simulink model "cube0_mpc_tp_ls"  (R2022b)
settings: Solver=VariableStepAuto  StartTime=0.0  StopTime=1000  RelTol=1e-3  AbsTol=1e-3
libraries: mpclib x1
settings Model: Creator=Abhijit  LastModifiedBy=Abhijit
settings SolverCC: AutoScaleAbsTol=off  AlgebraicLoopSolver=TrustRegion  MaxZcPerStep=1
settings DataIOCC: SaveFormat=StructureWithTime
settings DebuggingCC: UnconnectedInputMsg=warning  UnconnectedOutputMsg=warning  UnconnectedLineMsg=warning  SymbolicDimsDataTypeCodeGenerationDiagnostic=none  SFMachineParentedDataDiag=warning
settings ModelReferenceCC: EnableRefExpFcnMdlSchedulingChecks=on
settings SFSimCC: CustomCodeUndefinedFunction=UseInterfaceOnly
settings RTWCC: DLArmComputeVersion=19.05
settings SimscapeCC: SimscapeLogType=all  SimscapeLogSimulationStatistics=on  SimscapeLogDataHistory=10000

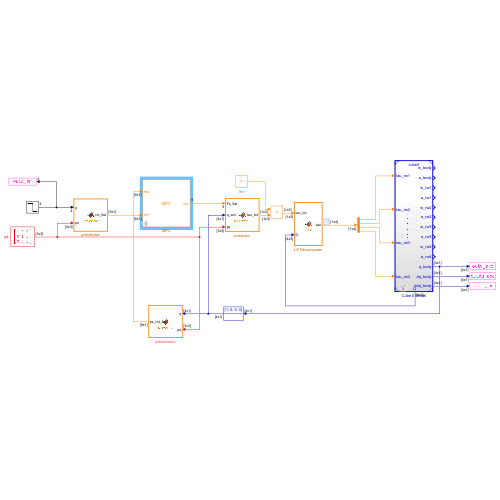
[thumbnail: Simulink's stored preview of the top-level diagram]
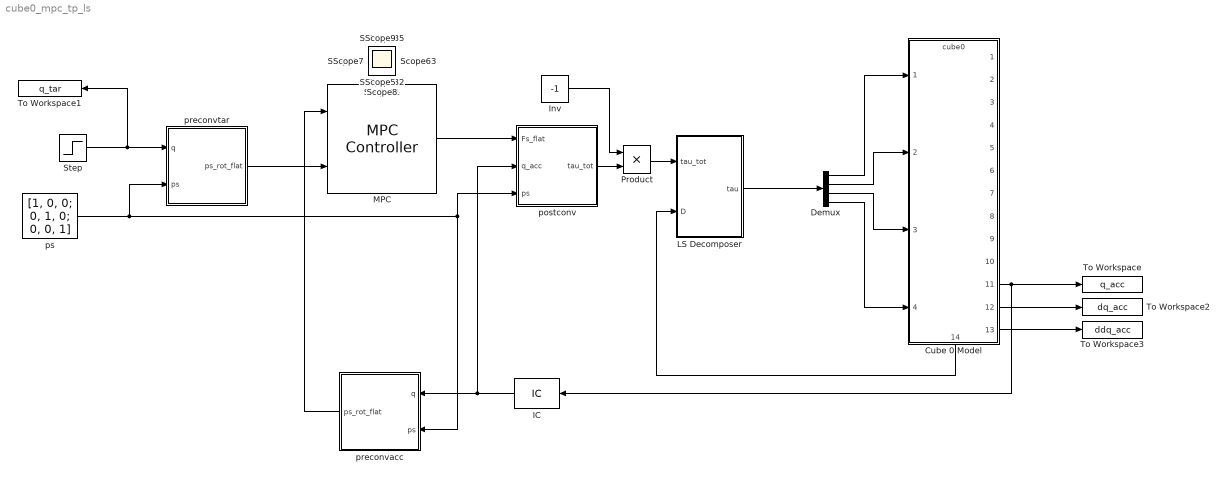
== system cube0_mpc_tp_ls ==
  Cube 0 Model : ModelReference  ModelNameDialog=cube0.slx  SimulationMode=Normal  ModelReferenceVersion=1.7
      settings: PortSchema="{\"entries\":[{\"content\":{\"sides\":[{\"content\":{\"connectorIds\":[\"In1\",\"In2\",\"In3\",\"In4\"]},\"type\":\"ConnectorPlacement.EquallySpacedRectSide\",\"uuid\":\"8e9d2764-0c8c-4b35-a6b5-330d2d8aade7\"},{\"content\":{\"connectorIds\":[\"Out1\",\"Out2\",\"Out3\",\"Out4\",\"Out5\",\"Out6\",\"Out7\",\"Out8\",\"Out9\",\"Out10\",\"Out11\",\"Out12\",\"Out13\"],\"side\":\"RIGHT\"},\"type\":\"ConnectorPlacement.EquallySpacedRectSide\",\"uuid\":\"d11583f7-9081-4803-9c4e-bf58094124c2\"},{\"content\":{\"connectorIds\":[],\"side\":\"TOP\"},\"type\":\"ConnectorPlacement.EquallySpacedRectSide\",\"uuid\":\"f987c09c-5813-428e-a812-016ca0940eea\"},{\"content\":{\"connectorIds\":[\"Out14\"],\"side\":\"BOTTOM\"},\"type\":\"ConnectorPlacement.EquallySpacedRectSide\",\"uuid\":\"56fa612c-373e-46c3-86f2-ebb8be87bff3\"}]},\"type\":\"ConnectorPlacement.EquallySpacedConnector\",\"uuid\":\"9c548295-d181-4ae3-baad-4641f0a6e641\"}],\"packageUris\":[\"http://schema.mathworks.com/mf0/Connector/R2020b\"],\"version\":\"1.0\"}"
  Demux : Demux
  IC : InitialCondition  Value=[1; 0; 0; 0]
  Inv : Constant  Value=-1
  LS Decomposer : MATLAB Function  TreatAsAtomicUnit=on
  MPC : mpclib/MPC Controller  SCDEnableBlockLinearizationSpecification=on  mpcobj=mpc1  is_multiple=0  enable_value=0  return_u0=off  updateMPCinCallerWorkspace=on  md_inport=off  mv_inport=off  uref_inport=off  return_cost=off  return_mvseq=off  return_qpstatus=off  return_xseq=off  return_state=off  return_ovseq=off  state_inport=off  umin_inport=off  umax_inport=off  ymin_inport=off  ymax_inport=off  cc_inport=off  ywt_inport=off  uwt_inport=off  duwt_inport=off  rhoeps_inport=off  pm_inport=off  MaximumP=10  HorizonChoice=FixedHorizon  n_ts=0.1  n_p=10  n_mv=9  n_md=0  n_ud=0  n_mo=9  n_uo=0  BlockDataType=double  SampleTimeInherited=off  switch_inport=off
  Product : Product
  Step : Step  Time=100  Before=[1 0 0 0]  After=[0.9981 0 0.043606 0.043606]  SampleTime=0
  To Workspace : ToWorkspace  VariableName=q_acc  SaveFormat=Timeseries  SampleTime=-1
  To Workspace1 : ToWorkspace  VariableName=q_tar  SaveFormat=Timeseries  SampleTime=-1
  To Workspace2 : ToWorkspace  VariableName=dq_acc  SaveFormat=Timeseries  SampleTime=-1
  To Workspace3 : ToWorkspace  VariableName=ddq_acc  SaveFormat=Timeseries  SampleTime=-1
  postconv : MATLAB Function  TreatAsAtomicUnit=on
  preconvacc : MATLAB Function  TreatAsAtomicUnit=on
      settings: MinAlgLoopOccurrences=on
  preconvtar : MATLAB Function  TreatAsAtomicUnit=on
  ps : Constant  Value=[1, 0, 0; 0, 1, 0; 0, 0, 1]
  Scope{,1..35} (36 alike) : Scope
  wires:
  Cube 0 Model/13 -> To Workspace3/1
  Cube 0 Model/12 -> To Workspace2/1
  Cube 0 Model/11 -> IC/1, To Workspace/1
  LS Decomposer/1(tau) -> Demux/1
  Demux/1 -> Cube 0 Model/1
  Demux/2 -> Cube 0 Model/2
  Demux/3 -> Cube 0 Model/3
  Demux/4 -> Cube 0 Model/4
  Cube 0 Model/14 -> LS Decomposer/2(D)
  preconvtar/1(ps_rot_flat) -> MPC/2
  Step/1 -> To Workspace1/1, preconvtar/1(q)
  ps/1 -> preconvtar/2(ps), preconvacc/2(ps), postconv/3(ps)
  MPC/1 -> postconv/1(Fs_flat)
  preconvacc/1(ps_rot_flat) -> MPC/1
  IC/1 -> postconv/2(q_acc), preconvacc/1(q)
  Product/1 -> LS Decomposer/1(tau_tot)
  postconv/1(tau_tot) -> Product/2
  Inv/1 -> Product/1

== matlab function cube0_mpc_tp_ls/LS Decomposer ==
  data: tau_tot input; tau output; D input
function tau = fcn(tau_tot, D)
    tau = lsdecomp(tau_tot, D);
end

== matlab function cube0_mpc_tp_ls/postconv ==
  data: Fs_flat input; q_acc input; tau_tot output; ps input
function tau_tot = postconv(Fs_flat, q_acc, ps)
    Fs = reshape(Fs_flat, 3, 3);
    qm_acc = quatconvert(q_acc, 'simulink', 'matlab');
    ps_acc = rotatepoint(qm_acc, ps);

    mn = size(ps_acc);
    taus = zeros(mn);
    for j = 1:mn(1)
        p_acc = ps_acc(j, :);
        F = Fs(j, :);
        taus(j, :) = cross(p_acc, F);
    end

    tau_tot = -1*sum(taus);
end

== matlab function cube0_mpc_tp_ls/preconvacc ==
  data: q input; ps_rot_flat output; ps input
function ps_rot_flat = preconv(q, ps)
    qm = quatconvert(q, 'simulink', 'matlab');
    ps_rot = rotatepoint(qm, ps);
    ps_rot_flat = reshape(ps_rot, 9, 1);
end

== matlab function cube0_mpc_tp_ls/preconvtar ==
  data: q input; ps_rot_flat output; ps input
function ps_rot_flat = preconv(q, ps)
    qm = quatconvert(q, 'simulink', 'matlab');
    ps_rot = rotatepoint(qm, ps);
    ps_rot_flat = reshape(ps_rot, 9, 1);
end
